simulink model "model_2"  (R2021a)
settings: Solver=VariableStepAuto  StartTime=0.0  StopTime=10.0  RelTol=1e-3
PreLoadFcn:
  | data
StopFcn:
  | drawing
CloseFcn:
  | drawing
settings Model: Creator=Beshary  LastModifiedBy=Beshary
settings DataIOCC: LoadExternalInput=on  SaveFormat=Array  InspectSignalLogs=on

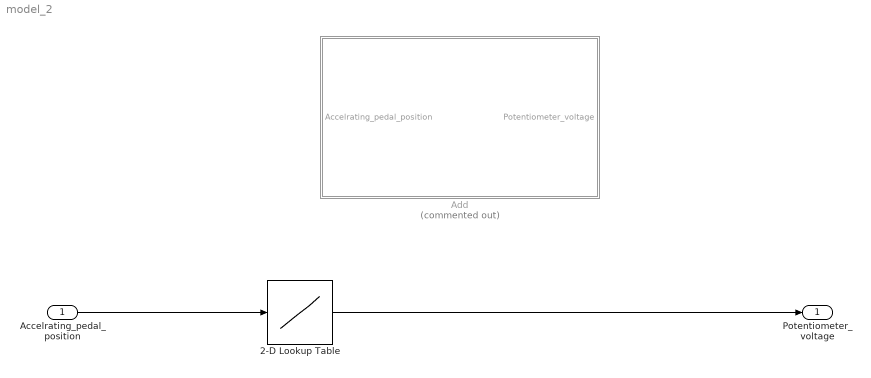
== system model_2 ==
  Accelrating_pedal_position : Inport
  2-D Lookup Table : Lookup_n-D  NumberOfTableDimensions=1  BreakpointsForDimension1=[0,0.1,0.2,0.3,0.4,0.5,0.6,0.7,0.8,0.9,1]  BreakpointsForDimension2=[1:3]  Table=[4.5,4.1,3.7,3.3,2.9,2.5,2.1,1.7,1.3,0.9,0.5]  InternalRulePriority=Speed  RndMeth=Simplest  InputSameDT=on
  Add : Subsystem  Commented=on
      mask DialogControl DescGroupVar Prompt: pedal
      mask DialogControl DescTextVar Prompt: pedal
      mask DialogControl Container4 Prompt: Tab
  Potentiometer_voltage : Outport
  wires:
  Accelrating_pedal_position/1 -> 2-D Lookup Table/1
  2-D Lookup Table/1 -> Potentiometer_voltage/1

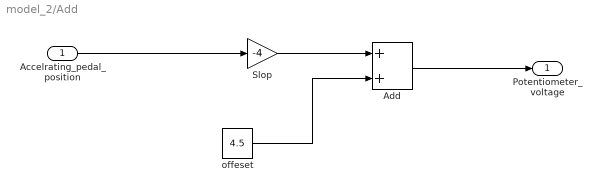
== system model_2/Add ==
  Accelrating_pedal_position : Inport
  Add : Sum
  Slop : Gain  Gain=-4
  offeset : Constant  Value=4.5
  Potentiometer_voltage : Outport
  wires:
  Accelrating_pedal_position/1 -> Slop/1
  Slop/1 -> Add/1
  offeset/1 -> Add/2
  Add/1 -> Potentiometer_voltage/1
